simulink model "test1_v2"  (R2018a)
settings: Solver=VariableStepAuto  StartTime=0.0  StopTime=100  FixedStep=0.01  RelTol=1e-3  EnableMultiTasking=on
InitFcn:
  | run constants
StopFcn:
  | run runafter
values from neighbouring files (symbols this model uses):
  F_0 = [0 0 0]    [constants2.m]
  phi_noise = noise_att_on * noise_att_mag    [constants2.m]
  pm_0 = [0 0 0]    [constants2.m]
  Psi_noise = noise_att_on * noise_att_mag    [constants2.m]
  R = (RE + 700*1000)    (= 7078000)    [constants2.m]
  T_d = Td_on * [0.001 0.001 0.001]    [constants2.m]
  theta_noise = noise_att_on * noise_att_mag    [constants2.m]
  Vm_0 = [0 Vc 0]    [constants2.m]
  xme_0 = [1 2 3]    [constants2.m]
undefined symbols (not defined in the file or in its folder): n
libraries: shared6dof x6, simulink x4, shared6dofsys x3, sharedutil x1, dspmathops x1
settings Model: PacingRate=1000  Creator=Matt  LastModifiedBy=matth
settings SolverCC: AutoInsertRateTranBlk=on
settings DataIOCC: SaveOutput=off  SaveTime=off
settings OptimizationCC: DefaultParameterBehavior=Inlined  InlineInvariantSignals=on  EnhancedBackFolding=on  PassReuseOutputArgsAs=Individual arguments  StateBitsets=on  DataBitsets=on  ZeroExternalMemoryAtStartup=off  ZeroInternalMemoryAtStartup=off  NoFixptDivByZeroProtection=on  LifeSpan=1  OptimizeBlockOrder=speed  DifferentSizesBufferReuse=on
settings DebuggingCC: ParameterTunabilityLossMsg=error
settings HardwareCC: ProdBitPerPointer=32  ProdBitPerSizeT=32  ProdBitPerPtrDiffT=32  ProdLargestAtomicFloat=None  ProdIntDivRoundTo=Floor  ProdWordSize=32  ProdHWDeviceType=Generic->Custom
settings SFSimCC: MATLABDynamicMemAlloc=off
settings RTWCC: SystemTargetFile=ert.tlc  TLCOptions=-p0  GenCodeOnly=on  TemplateMakefile=ert_default_tmf  GenerateReport=on  RTWVerbose=off  IncludeHyperlinkInReport=on  LaunchReport=on  GenerateTraceInfo=on  GenerateTraceReport=on  GenerateTraceReportSl=on  GenerateTraceReportSf=on  GenerateTraceReportEml=on
settings CodeAppCC: ForceParamTrailComments=on  IgnoreCustomStorageClasses=off  OperatorAnnotations=on  SimulinkDataObjDesc=on  SFDataObjDesc=on  CustomSymbolStrGlobalVar=rt$N$M  CustomSymbolStrType=$N$M  CustomSymbolStrFcn=$N$M$F  CustomSymbolStrMacro=$N$M  InsertBlockDesc=on
settings ERTTargetCC: TargetLangStandard=C99 (ISO)  CodeReplacementLibrary=ISO_C  GenerateSampleERTMain=on  IncludeMdlTerminateFcn=off  SuppressErrorStatus=on  SupportAbsoluteTime=off  SupportNonFinite=off  SupportComplex=off  PurelyIntegerCode=on  InlinedParameterPlacement=NonHierarchical  RootIOFormat=Structure reference  ERTCustomFileTemplate=example_file_process.tlc

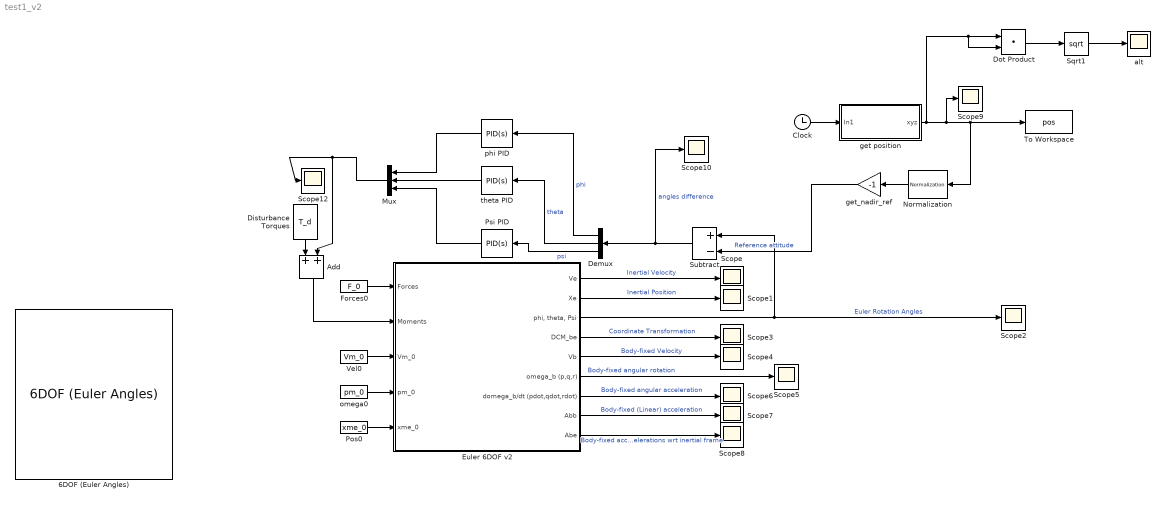
== system test1_v2 ==
  6DOF (Euler Angles) : shared6dof/6DOF (Euler Angles)  units=Metric (MKS)  mtype=Fixed  rep=Euler Angles  xme_0=[0 0 0]  Vm_0=[0 0 0]  eul_0=[0 0 0]  pm_0=[0 0 0]  mass_0=1.0  mass_e=0.5  mass_f=2.0  inertia=eye(3)  inertia_e=eye(3)  inertia_f=2*eye(3)  k_quat=1.0  vre_flag=on  abi_flag=off  aMode=0
      settings: SourceProductBaseCode=AE
  Add : Sum
  Clock : Clock
  Demux : Demux  Outputs=3
  Disturbance Torques : Constant  Value=T_d
  Dot Product : DotProduct  InputSameDT=on  OutDataTypeStr=Inherit: Inherit via internal rule
  Euler 6DOF v2 : Subsystem
  Forces0 : Constant  Value=F_0
  Mux : Mux  Inputs=3
  Normalization : dspmathops/Normalization  NormType=2-norm  Bias=1e-10  NormOver=Each column  Dimension=1  roundingMode=Floor  overflowMode=off  accumDataTypeStr=Inherit: Same as product output  accumLastDataTypeStr=Inherit: Same as product output  outputDataTypeStr=Inherit: Same as product output  outputMin=[]  outputMax=[]  outputLastDataTypeStr=Inherit: Same as product output
      settings: SourceProductName=DSP System Toolbox
  Pos0 : Constant  Value=xme_0
  Psi PID : simulink/Continuous/PID Controller  Controller=PID  TimeDomain=Continuous-time  SampleTime=-1  IntegratorMethod=Forward Euler  FilterMethod=Forward Euler  Form=Parallel  UseFilter=on  ControllerParametersSource=internal  P=-730.157338378478  I=-36.609264068618  D=-2842.71233291057  N=10.4897155810233  InitialConditionSource=internal  InitialConditionForIntegrator=0  InitialConditionForFilter=0  ExternalReset=none  LimitOutput=off  UpperSaturationLimit=inf  LowerSaturationLimit=-inf  LinearizeAsGain=on  AntiWindupMode=none  Kb=1  TrackingMode=off  Kt=1  PParamMin=[]  PParamMax=[]  IParamMin=[]  IParamMax=[]  DParamMin=[]  DParamMax=[]  NParamMin=[]  NParamMax=[]  KbParamMin=[]  KbParamMax=[]  KtParamMin=[]  KtParamMax=[]  POutMin=[]  POutMax=[]  IOutMin=[]  IOutMax=[]  DOutMin=[]  DOutMax=[]  NOutMin=[]  NOutMax=[]  KbOutMin=[]  KbOutMax=[]  KtOutMin=[]  KtOutMax=[]  IntegratorOutMin=[]  IntegratorOutMax=[]  FilterOutMin=[]  FilterOutMax=[]  SumOutMin=[]  SumOutMax=[]  SumI1OutMin=[]  SumI1OutMax=[]  SumI2OutMin=[]  SumI2OutMax=[]  SumI3OutMin=[]  SumI3OutMax=[]  SumDOutMin=[]  SumDOutMax=[]  SaturationOutMin=[]  SaturationOutMax=[]  IntegratorContinuousStateAttributes=''  IntegratorStateMustResolveToSignalObject=off  IntegratorRTWStateStorageClass=Auto  FilterContinuousStateAttributes=''  FilterStateMustResolveToSignalObject=off  FilterRTWStateStorageClass=Auto  DifferentiatorICPrevScaledInput=0  DifferentiatorOutMin=[]  DifferentiatorOutMax=[]  FilterDiffOutCoefMin=[]  FilterDiffOutCoefMax=[]  SumDenOutMin=[]  SumDenOutMax=[]  SumNumOutMin=[]  SumNumOutMax=[]  ReciprocalOutMin=[]  ReciprocalOutMax=[]  DivideOutMin=[]  DivideOutMax=[]  TunerSelectOption=Transfer Function Based (PID Tuner App)
  Scope{,1..10,12} (12 alike) : Scope
  Sqrt1 : Sqrt  SaturateOnIntegerOverflow=on
  Subtract : Sum  Inputs=+-
  To Workspace : ToWorkspace  VariableName=pos  SaveFormat=Timeseries  SampleTime=-1
  Vel0 : Constant  Value=Vm_0
  alt : Scope
  get position : Subsystem
  "get_nadir_ref " : Gain  Gain=-1
  "omega0 " : Constant  Value=pm_0
  "phi PID " : simulink/Continuous/PID Controller  Controller=PID  TimeDomain=Continuous-time  SampleTime=-1  IntegratorMethod=Forward Euler  FilterMethod=Forward Euler  Form=Parallel  UseFilter=on  ControllerParametersSource=internal  P=-464.198158177747  I=-21.7313338529705  D=-2434.80245399495  N=5.45397025421619  InitialConditionSource=internal  InitialConditionForIntegrator=0  InitialConditionForFilter=0  ExternalReset=none  LimitOutput=off  UpperSaturationLimit=inf  LowerSaturationLimit=-inf  LinearizeAsGain=on  AntiWindupMode=none  Kb=1  TrackingMode=off  Kt=1  PParamMin=[]  PParamMax=[]  IParamMin=[]  IParamMax=[]  DParamMin=[]  DParamMax=[]  NParamMin=[]  NParamMax=[]  KbParamMin=[]  KbParamMax=[]  KtParamMin=[]  KtParamMax=[]  POutMin=[]  POutMax=[]  IOutMin=[]  IOutMax=[]  DOutMin=[]  DOutMax=[]  NOutMin=[]  NOutMax=[]  KbOutMin=[]  KbOutMax=[]  KtOutMin=[]  KtOutMax=[]  IntegratorOutMin=[]  IntegratorOutMax=[]  FilterOutMin=[]  FilterOutMax=[]  SumOutMin=[]  SumOutMax=[]  SumI1OutMin=[]  SumI1OutMax=[]  SumI2OutMin=[]  SumI2OutMax=[]  SumI3OutMin=[]  SumI3OutMax=[]  SumDOutMin=[]  SumDOutMax=[]  SaturationOutMin=[]  SaturationOutMax=[]  IntegratorContinuousStateAttributes=''  IntegratorStateMustResolveToSignalObject=off  IntegratorRTWStateStorageClass=Auto  FilterContinuousStateAttributes=''  FilterStateMustResolveToSignalObject=off  FilterRTWStateStorageClass=Auto  DifferentiatorICPrevScaledInput=0  DifferentiatorOutMin=[]  DifferentiatorOutMax=[]  FilterDiffOutCoefMin=[]  FilterDiffOutCoefMax=[]  SumDenOutMin=[]  SumDenOutMax=[]  SumNumOutMin=[]  SumNumOutMax=[]  ReciprocalOutMin=[]  ReciprocalOutMax=[]  DivideOutMin=[]  DivideOutMax=[]  TunerSelectOption=Transfer Function Based (PID Tuner App)
  theta PID : simulink/Continuous/PID Controller  Controller=PID  TimeDomain=Continuous-time  SampleTime=-1  IntegratorMethod=Forward Euler  FilterMethod=Forward Euler  Form=Parallel  UseFilter=on  ControllerParametersSource=internal  P=-568.423410964435  I=-28.5001924417647  D=-2213.03320065217  N=10.4897155810233  InitialConditionSource=internal  InitialConditionForIntegrator=0  InitialConditionForFilter=0  ExternalReset=none  LimitOutput=off  UpperSaturationLimit=inf  LowerSaturationLimit=-inf  LinearizeAsGain=on  AntiWindupMode=none  Kb=1  TrackingMode=off  Kt=1  PParamMin=[]  PParamMax=[]  IParamMin=[]  IParamMax=[]  DParamMin=[]  DParamMax=[]  NParamMin=[]  NParamMax=[]  KbParamMin=[]  KbParamMax=[]  KtParamMin=[]  KtParamMax=[]  POutMin=[]  POutMax=[]  IOutMin=[]  IOutMax=[]  DOutMin=[]  DOutMax=[]  NOutMin=[]  NOutMax=[]  KbOutMin=[]  KbOutMax=[]  KtOutMin=[]  KtOutMax=[]  IntegratorOutMin=[]  IntegratorOutMax=[]  FilterOutMin=[]  FilterOutMax=[]  SumOutMin=[]  SumOutMax=[]  SumI1OutMin=[]  SumI1OutMax=[]  SumI2OutMin=[]  SumI2OutMax=[]  SumI3OutMin=[]  SumI3OutMax=[]  SumDOutMin=[]  SumDOutMax=[]  SaturationOutMin=[]  SaturationOutMax=[]  IntegratorContinuousStateAttributes=''  IntegratorStateMustResolveToSignalObject=off  IntegratorRTWStateStorageClass=Auto  FilterContinuousStateAttributes=''  FilterStateMustResolveToSignalObject=off  FilterRTWStateStorageClass=Auto  DifferentiatorICPrevScaledInput=0  DifferentiatorOutMin=[]  DifferentiatorOutMax=[]  FilterDiffOutCoefMin=[]  FilterDiffOutCoefMax=[]  SumDenOutMin=[]  SumDenOutMax=[]  SumNumOutMin=[]  SumNumOutMax=[]  ReciprocalOutMin=[]  ReciprocalOutMax=[]  DivideOutMin=[]  DivideOutMax=[]  TunerSelectOption=Transfer Function Based (PID Tuner App)
  wires:
  Euler 6DOF v2/1(Ve) -> Scope/1  "Inertial Velocity"
  Euler 6DOF v2/2(Xe) -> Scope1/1  "Inertial Position"
  Euler 6DOF v2/3("phi, theta, Psi") -> Subtract/1, Scope2/1  "Euler Rotation Angles"
  Euler 6DOF v2/4(DCM_be) -> Scope3/1  "Coordinate Transformation"
  Euler 6DOF v2/5(Vb) -> Scope4/1  "Body-fixed Velocity"
  Euler 6DOF v2/6(omega_b (p,q,r)) -> Scope5/1  "Body-fixed angular rotation"
  Euler 6DOF v2/7(domega_b/dt (pdot,qdot,rdot)) -> Scope6/1  "Body-fixed angular acceleration"
  Euler 6DOF v2/8(Abb) -> Scope7/1  "Body-fixed (Linear) acceleration"
  Euler 6DOF v2/9(Abe) -> Scope8/1  "Body-fixed accelerations wrt inertial frame"
  "get_nadir_ref "/1 -> Subtract/2  "Reference attitude"
  Demux/1 -> "phi PID "/1  "phi"
  Demux/2 -> theta PID/1  "theta"
  Demux/3 -> Psi PID/1  "psi"
  "phi PID "/1 -> Mux/1
  theta PID/1 -> Mux/2
  Psi PID/1 -> Mux/3
  Mux/1 -> Add/2, Scope12/1
  Subtract/1 -> Scope10/1, Demux/1  "angles difference"
  Forces0/1 -> Euler 6DOF v2/1(Forces)
  Vel0/1 -> Euler 6DOF v2/3(Vm_0)
  Pos0/1 -> Euler 6DOF v2/5("xme_0 ")
  "omega0 "/1 -> Euler 6DOF v2/4("pm_0 ")
  Disturbance Torques/1 -> Add/1
  Add/1 -> Euler 6DOF v2/2(Moments)
  Dot Product/1 -> Sqrt1/1
  Sqrt1/1 -> alt/1
  Clock/1 -> get position/1(In1)
  get position/1(xyz) -> Dot Product/2, Dot Product/1, Normalization/1, To Workspace/1, Scope9/1
  Normalization/1 -> "get_nadir_ref "/1

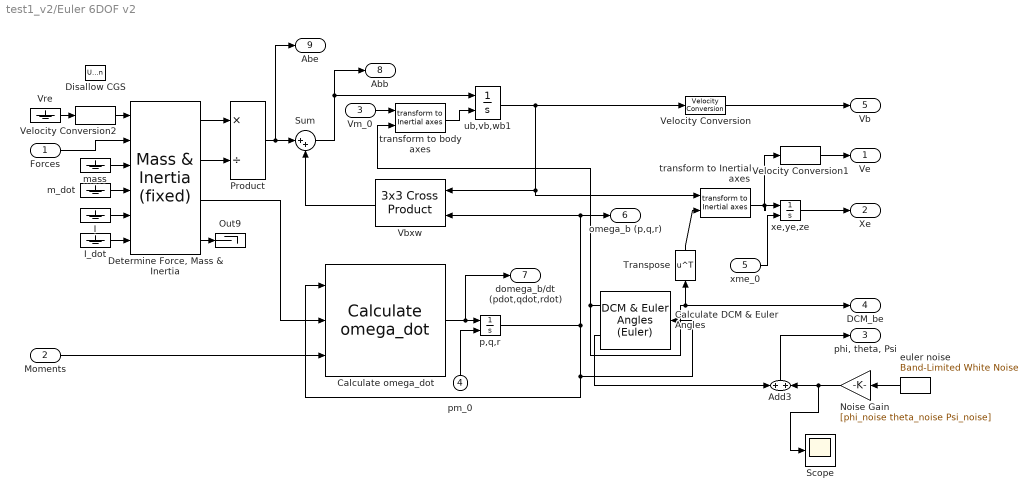
== system test1_v2/Euler 6DOF v2 ==
  Forces : Inport  Unit=N  PortDimensions=3
  Moments : Inport  Port=2  Unit=N*m  PortDimensions=3
  Vm_0 : Inport  Port=3
  "pm_0 " : Inport  Port=4
  "xme_0 " : Inport  Port=5
  Add3 : Sum
  Calculate DCM & Euler Angles : shared6dofsys/DCM & Euler Angles (Euler)  aMode=aMode
      settings: SourceProductName=Aerospace Blockset  SourceProductBaseCode=AE
  Calculate omega_dot : shared6dofsys/Calculate omega_dot  aMode=aMode
      settings: SourceProductName=Aerospace Blockset  SourceProductBaseCode=AE
  "Determine Force, Mass & Inertia" : shared6dofsys/Mass & Inertia (fixed)  aMode=aMode
      settings: SourceProductName=Aerospace Blockset  SourceProductBaseCode=AE
  Disallow CGS : UnitConfiguration  UnitSystemsStr=English,SI,SI (extended)  AllowAllUnitSystems=off
  I : Ground
  I_dot : Ground
  Noise Gain : Gain  Gain=[phi_noise theta_noise Psi_noise]
  Out9 : Terminator
  Product : Product  Inputs=*/  SaturateOnIntegerOverflow=on  OutDataTypeStr=Inherit: Same as first input
  Scope : Scope
  Sum : Sum  Inputs=|++  SaturateOnIntegerOverflow=on
  Transpose : Math  Operator=transpose  SaturateOnIntegerOverflow=on
  Vbxw : sharedutil/3x3 Cross Product  aMode=aMode
      settings: SourceProductBaseCode=AE
  Velocity Conversion : shared6dof/6DOF (Euler Angles)/Velocity Conversion
      settings: SourceProductName=Aerospace Blockset  SourceProductBaseCode=AE
  Velocity Conversion1 : shared6dof/6DOF (Euler Angles)/Velocity Conversion1
      settings: SourceProductName=Aerospace Blockset  SourceProductBaseCode=AE
  Velocity Conversion2 : shared6dof/6DOF (Euler Angles)/Velocity Conversion2
      settings: SourceProductName=Aerospace Blockset  SourceProductBaseCode=AE
  Vre : Ground
  euler noise : simulink/Sources/Band-Limited White Noise  Cov=[0.1]  Ts=1  seed=[23341]
  m_dot : Ground
  mass : Ground
  "p,q,r " : Integrator  InitialConditionSource=external  InitialCondition=pm_0
  "transform to Inertial axes " : shared6dof/6DOF (Euler Angles)/transform to Inertial axes   SystemSampleTime=-1
      settings: SourceProductName=Aerospace Blockset  SourceProductBaseCode=AE
  transform to body axes : shared6dof/6DOF (Euler Angles)/transform to Inertial axes   SystemSampleTime=-1
      settings: SourceProductName=Aerospace Blockset  SourceProductBaseCode=AE
  ub,vb,wb1 : Integrator  InitialConditionSource=external  InitialCondition=Vm_0
  xe,ye,ze : Integrator  InitialConditionSource=external  InitialCondition=xme_0
  Ve : Outport  Unit=m/s
  Xe : Outport  Port=2  Unit=m
  "phi, theta, Psi" : Outport  Port=3  Unit=rad
  DCM_be : Outport  Port=4  Unit=1
  Vb : Outport  Port=5  Unit=m/s
  omega_b (p,q,r) : Outport  Port=6  Unit=rad/s
  domega_b/dt (pdot,qdot,rdot) : Outport  Port=7  Unit=rad/s^2
  Abb : Outport  Port=8  Unit=m/s^2
  Abe : Outport  Port=9  Unit=m/s^2
  wires:
  Calculate DCM & Euler Angles/1 -> transform to body axes/2, Transpose/1, DCM_be/1
  Vbxw/1 -> Sum/2
  Velocity Conversion/1 -> Vb/1
  xe,ye,ze/1 -> Xe/1
  Vre/1 -> Velocity Conversion2/1
  Calculate DCM & Euler Angles/2 -> Add3/1
  "p,q,r "/1 -> Calculate omega_dot/1, Calculate DCM & Euler Angles/1, omega_b (p,q,r)/1, Vbxw/2
  Product/1 -> Sum/1, Abe/1
  Moments/1 -> Calculate omega_dot/3
  "Determine Force, Mass & Inertia"/2 -> Product/2
  "transform to Inertial axes "/1 -> xe,ye,ze/1, Velocity Conversion1/1
  "Determine Force, Mass & Inertia"/4 -> Out9/1
  Transpose/1 -> "transform to Inertial axes "/2
  mass/1 -> "Determine Force, Mass & Inertia"/3
  Velocity Conversion1/1 -> Ve/1
  Calculate omega_dot/1 -> "p,q,r "/1, domega_b/dt (pdot,qdot,rdot)/1
  I/1 -> "Determine Force, Mass & Inertia"/5
  "Determine Force, Mass & Inertia"/3 -> Calculate omega_dot/2
  ub,vb,wb1/1 -> "transform to Inertial axes "/1, Vbxw/1, Velocity Conversion/1
  "Determine Force, Mass & Inertia"/1 -> Product/1
  Forces/1 -> "Determine Force, Mass & Inertia"/2
  Velocity Conversion2/1 -> "Determine Force, Mass & Inertia"/1
  I_dot/1 -> "Determine Force, Mass & Inertia"/6
  Sum/1 -> Abb/1, ub,vb,wb1/1
  m_dot/1 -> "Determine Force, Mass & Inertia"/4
  Vm_0/1 -> transform to body axes/1
  "pm_0 "/1 -> "p,q,r "/2
  "xme_0 "/1 -> xe,ye,ze/2
  Noise Gain/1 -> Scope/1, Add3/2
  Add3/1 -> "phi, theta, Psi"/1
  euler noise/1 -> Noise Gain/1
  transform to body axes/1 -> ub,vb,wb1/2

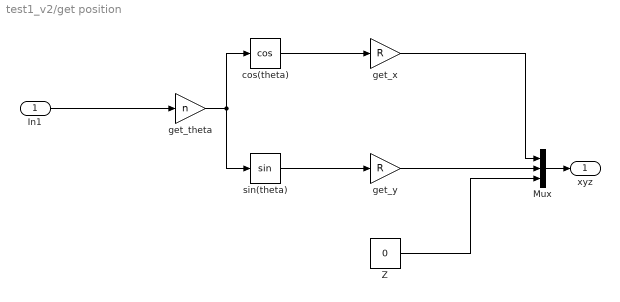
== system test1_v2/get position ==
  In1 : Inport
  Mux : Mux  Inputs=3
  "Z " : Constant  Value=0
  cos(theta) : Trigonometry  Operator=cos
  get_theta : Gain  Gain=n
  "get_x " : Gain  Gain=R
  get_y : Gain  Gain=R
  sin(theta) : Trigonometry
  xyz : Outport
  wires:
  In1/1 -> get_theta/1
  get_theta/1 -> cos(theta)/1, sin(theta)/1
  cos(theta)/1 -> "get_x "/1
  sin(theta)/1 -> get_y/1
  "Z "/1 -> Mux/3
  get_y/1 -> Mux/2
  "get_x "/1 -> Mux/1
  Mux/1 -> xyz/1
